simulink model "Enabled1_2018a"  (R2018a)
settings: Solver=VariableStepAuto  StartTime=0.0  StopTime=20  RelTol=1e-3
settings Model: Creator=BEAR  LastModifiedBy=bzhan

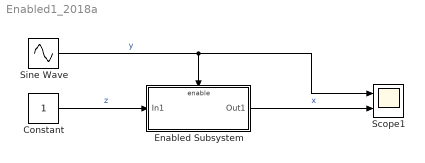
== system Enabled1_2018a ==
  Constant : Constant
  Enabled Subsystem : Subsystem  TreatAsAtomicUnit=on
  Scope1 : Scope  NumInputPorts=2
  Sine Wave : Sin  SampleTime=0
  wires:
  Sine Wave/1 -> Scope1/1, Enabled Subsystem/Enable  "y"
  Constant/1 -> Enabled Subsystem/1(In1)  "z"
  Enabled Subsystem/1(Out1) -> Scope1/2  "x"

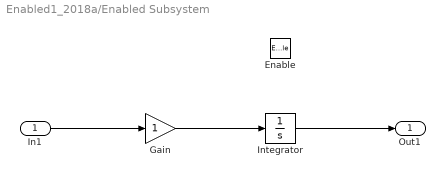
== system Enabled1_2018a/Enabled Subsystem ==
  In1 : Inport
  Enable : EnablePort
  Gain : Gain  SampleTime=2
  Integrator : Integrator
  Out1 : Outport  VectorParamsAs1DForOutWhenUnconnected=off
  wires:
  Integrator/1 -> Out1/1
  In1/1 -> Gain/1
  Gain/1 -> Integrator/1
